simulink model "Virtual_Fuel_Air_Setpoint_Generator"  (R2016b)
settings: Solver=FixedStepDiscrete  StartTime=0.0  StopTime=inf  FixedStep=VirtFuAirSpGenr.tiSimnTiStep_C  RelTol=1e-3  EnableMultiTasking=on
settings Model: Creator=m01wolf  LastModifiedBy=bunver
settings DataIOCC: SaveFormat=StructureWithTime  SaveOutput=off  DSMLogging=off  VisualizeSimOutput=off  SaveTime=off  StateSaveName=Results  SignalLoggingName=Results
settings OptimizationCC: BlockReduction=off  ConditionallyExecuteInputs=off  LifeSpan=inf
settings DebuggingCC: AllowSymbolicDim=off  SFUnexpectedBacktrackingDiag=warning  SFNoUnconditionalDefaultTransitionDiag=warning  SFExecutionAtInitializationDiag=none
settings ModelReferenceCC: ModelReferenceNumInstancesAllowed=Single  PropagateSignalLabelsOutOfModel=off
settings GRTTargetCC: TargetLangStandard=C89/C90 (ANSI)
settings ConfigComp: CovMetricSettings=dw  CovHtmlReporting=on  CovSaveCumulativeToWorkspaceVar=on  CovSaveSingleToWorkspaceVar=on  CovExternalEMLEnable=off

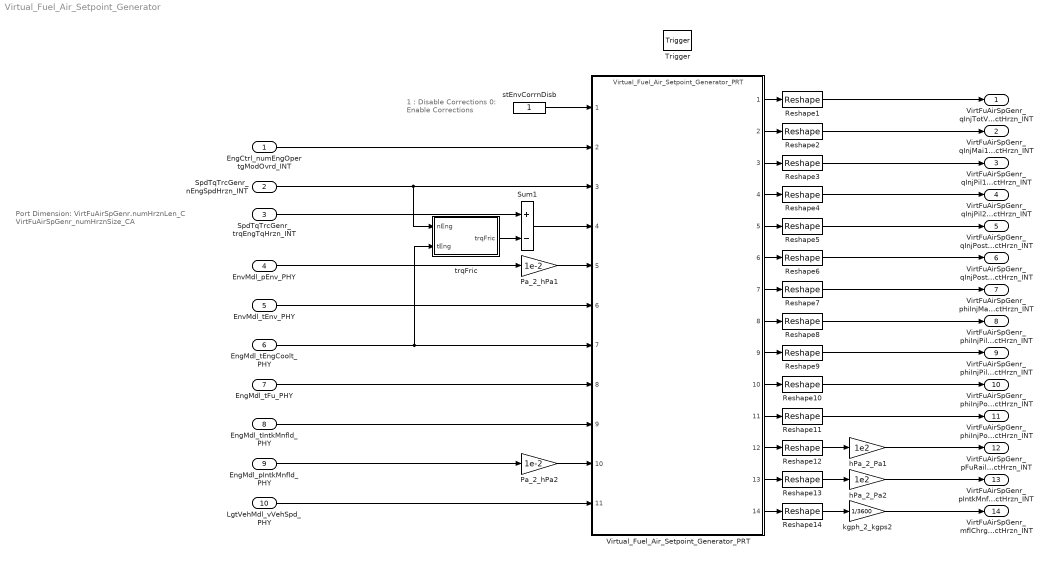
== system Virtual_Fuel_Air_Setpoint_Generator ==
  note: Port Dimension: VirtFuAirSpGenr.numHrznLen_C
      | VirtFuAirSpGenr_numHrznSize_CA
  note: 1 : Disable Corrections
      | 0: Enable Corrections
  EngCtrl_numEngOpertgModOvrd_INT : Inport
  SpdTqTrcGenr_nEngSpdHrzn_INT : Inport  Port=2  PortDimensions=VirtFuAirSpGenr_numHrznSize_CA
  SpdTqTrcGenr_trqEngTqHrzn_INT : Inport  Port=3  PortDimensions=VirtFuAirSpGenr_numHrznSize_CA
  EnvMdl_pEnv_PHY : Inport  Port=4
  EnvMdl_tEnv_PHY : Inport  Port=5
  EngMdl_tEngCoolt_PHY : Inport  Port=6
  EngMdl_tFu_PHY : Inport  Port=7
  EngMdl_tIntkMnfld_PHY : Inport  Port=8
  EngMdl_pIntkMnfld_PHY : Inport  Port=9
  LgtVehMdl_vVehSpd_PHY : Inport  Port=10
  Trigger : TriggerPort  TriggerType=function-call  VariantControl=Variant  PortDimensions=1
  Pa_2_hPa1 : Gain  Gain=1e-2
  Pa_2_hPa2 : Gain  Gain=1e-2
  Reshape{1..14} (14 alike) : Reshape
  Sum1 : Sum  Inputs=+-
      settings: AttributesFormatString=%<Name>
  Virtual_Fuel_Air_Setpoint_Generator_PRT : ModelReference  ModelNameDialog=Virtual_Fuel_Air_Setpoint_Generator_PRT.slxp  ModelReferenceVersion=1.262  CopyOfModelProtected=on
  hPa_2_Pa1 : Gain  Gain=1e2
  hPa_2_Pa2 : Gain  Gain=1e2
  kgph_2_kgps2 : Gain  Gain=1/3600
  stEnvCorrnDisb : Constant  SampleTime=-1
  trqFric : Subsystem
  VirtFuAirSpGenr_qInjTotVectHrzn_INT : Outport
  VirtFuAirSpGenr_qInjMai1VectHrzn_INT : Outport  Port=2
  VirtFuAirSpGenr_qInjPil1VectHrzn_INT : Outport  Port=3
  VirtFuAirSpGenr_qInjPil2VectHrzn_INT : Outport  Port=4
  VirtFuAirSpGenr_qInjPost1VectHrzn_INT : Outport  Port=5
  VirtFuAirSpGenr_qInjPost2VectHrzn_INT : Outport  Port=6
  VirtFuAirSpGenr_phiInjMai1VectHrzn_INT : Outport  Port=7
  VirtFuAirSpGenr_phiInjPil1VectHrzn_INT : Outport  Port=8
  VirtFuAirSpGenr_phiInjPil2VectHrzn_INT : Outport  Port=9
  VirtFuAirSpGenr_phiInjPost1VectHrzn_INT : Outport  Port=10
  VirtFuAirSpGenr_phiInjPost2VectHrzn_INT : Outport  Port=11
  VirtFuAirSpGenr_pFuRailDesVectHrzn_INT : Outport  Port=12
  VirtFuAirSpGenr_pIntkMnfldDesVectHrzn_INT : Outport  Port=13
  VirtFuAirSpGenr_mflChrgdAirDesVectHrzn_INT : Outport  Port=14
  wires:
  Virtual_Fuel_Air_Setpoint_Generator_PRT/1 -> Reshape1/1
  hPa_2_Pa1/1 -> VirtFuAirSpGenr_pFuRailDesVectHrzn_INT/1
  hPa_2_Pa2/1 -> VirtFuAirSpGenr_pIntkMnfldDesVectHrzn_INT/1
  kgph_2_kgps2/1 -> VirtFuAirSpGenr_mflChrgdAirDesVectHrzn_INT/1
  Virtual_Fuel_Air_Setpoint_Generator_PRT/2 -> Reshape2/1
  Virtual_Fuel_Air_Setpoint_Generator_PRT/3 -> Reshape3/1
  Virtual_Fuel_Air_Setpoint_Generator_PRT/4 -> Reshape4/1
  Virtual_Fuel_Air_Setpoint_Generator_PRT/5 -> Reshape5/1
  Virtual_Fuel_Air_Setpoint_Generator_PRT/6 -> Reshape6/1
  Virtual_Fuel_Air_Setpoint_Generator_PRT/7 -> Reshape7/1
  Virtual_Fuel_Air_Setpoint_Generator_PRT/8 -> Reshape8/1
  Virtual_Fuel_Air_Setpoint_Generator_PRT/9 -> Reshape9/1
  Virtual_Fuel_Air_Setpoint_Generator_PRT/10 -> Reshape10/1
  Virtual_Fuel_Air_Setpoint_Generator_PRT/11 -> Reshape11/1
  Virtual_Fuel_Air_Setpoint_Generator_PRT/12 -> Reshape12/1
  Virtual_Fuel_Air_Setpoint_Generator_PRT/13 -> Reshape13/1
  Virtual_Fuel_Air_Setpoint_Generator_PRT/14 -> Reshape14/1
  trqFric/1(trqFric) -> Sum1/2
  Reshape1/1 -> VirtFuAirSpGenr_qInjTotVectHrzn_INT/1
  Reshape2/1 -> VirtFuAirSpGenr_qInjMai1VectHrzn_INT/1
  Reshape3/1 -> VirtFuAirSpGenr_qInjPil1VectHrzn_INT/1
  Reshape4/1 -> VirtFuAirSpGenr_qInjPil2VectHrzn_INT/1
  Reshape5/1 -> VirtFuAirSpGenr_qInjPost1VectHrzn_INT/1
  Reshape6/1 -> VirtFuAirSpGenr_qInjPost2VectHrzn_INT/1
  Reshape7/1 -> VirtFuAirSpGenr_phiInjMai1VectHrzn_INT/1
  Reshape8/1 -> VirtFuAirSpGenr_phiInjPil1VectHrzn_INT/1
  Reshape9/1 -> VirtFuAirSpGenr_phiInjPil2VectHrzn_INT/1
  Reshape10/1 -> VirtFuAirSpGenr_phiInjPost1VectHrzn_INT/1
  Reshape11/1 -> VirtFuAirSpGenr_phiInjPost2VectHrzn_INT/1
  Reshape12/1 -> hPa_2_Pa1/1
  Reshape13/1 -> hPa_2_Pa2/1
  Reshape14/1 -> kgph_2_kgps2/1
  SpdTqTrcGenr_nEngSpdHrzn_INT/1 -> Virtual_Fuel_Air_Setpoint_Generator_PRT/3, trqFric/1(nEng)
  SpdTqTrcGenr_trqEngTqHrzn_INT/1 -> Sum1/1
  EnvMdl_pEnv_PHY/1 -> Pa_2_hPa1/1
  EngMdl_tEngCoolt_PHY/1 -> Virtual_Fuel_Air_Setpoint_Generator_PRT/7, trqFric/2(tEng)
  EngMdl_pIntkMnfld_PHY/1 -> Pa_2_hPa2/1
  stEnvCorrnDisb/1 -> Virtual_Fuel_Air_Setpoint_Generator_PRT/1
  EngCtrl_numEngOpertgModOvrd_INT/1 -> Virtual_Fuel_Air_Setpoint_Generator_PRT/2
  Sum1/1 -> Virtual_Fuel_Air_Setpoint_Generator_PRT/4
  Pa_2_hPa1/1 -> Virtual_Fuel_Air_Setpoint_Generator_PRT/5
  EnvMdl_tEnv_PHY/1 -> Virtual_Fuel_Air_Setpoint_Generator_PRT/6
  EngMdl_tFu_PHY/1 -> Virtual_Fuel_Air_Setpoint_Generator_PRT/8
  EngMdl_tIntkMnfld_PHY/1 -> Virtual_Fuel_Air_Setpoint_Generator_PRT/9
  Pa_2_hPa2/1 -> Virtual_Fuel_Air_Setpoint_Generator_PRT/10
  LgtVehMdl_vVehSpd_PHY/1 -> Virtual_Fuel_Air_Setpoint_Generator_PRT/11

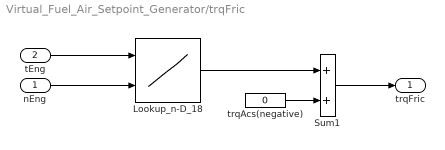
== system Virtual_Fuel_Air_Setpoint_Generator/trqFric ==
  nEng : Inport
  tEng : Inport  Port=2
  Lookup_n-D_18 : Lookup_n-D  BreakpointsForDimension1=[-30.14;-20.14;-10.14;-0.140000000000009;9.85999999999999;19.86;29.86;39.86;49.86;59.86;69.86;79.86;89.86;99.86;109.86;119.86]  BreakpointsForDimension2=[600 700 800 900 1000 1100 1200 1300 1400 1500 1600 1700 1800 1900 2000 2100]  Table=[-490 -505 -515 -520 -530 -540 -545 -550 -555 -560 -565 -570 -575 -580 -590 -600;-490 -505 -515 -520 -530 -540 -545 -550 -555 -560 -565 -570 -575 -580 -590 -600;-420 -427 -431 -433 -435 -437 -441.333343505859 -445.666656494141 -450 -455 -460 -465 -470 -500 -515 -524;-250 -277.5 -305 -309 -311 -316 -324 -335 -345 -352 -365 -379 -397 -410 -425 -450;-234 -249.25 -266.5 -271 -274 -283 -293.904754638672 -306.309509277344 -318.214294433594 -330 -342.023803710938 -355.928588867188 -370 -392.75 -415.5 -436.75;-218 -221 -228 -233 -237 -250 -263.809509277344 -277.619049072266 -291.428558349609 -304 -319.047607421875 -332.857147216797 -346.666656494141 -372.375 -393 -413.5;-199.5 -201.5 -208.5 -213 -217.5 -230 -242.904754638672 -256.809509277344 -270.714294433594 -284.619049072266 -297.523803710938 -310.928588867188 -323.333343505859 -352 -370.5 -390.25;-181 -182 -189 -193 -198 -210 -222 -236 -250 -264 -276 -289 -300 -329 -348 -367;-138 -149.199996948242 -159.399993896484 -170 -181.100006103516 -192.600006103516 -204.899993896484 -222 -236.100006103516 -246.899993896484 -263.600006103516 -277.5 -286.100006103516 -297.200012207031 -325.700012207031 -344.899993896484;-129 -138.300003051758 -147.699996948242 -157.800003051758 -168.100006103516 -179.600006103516 -191.100006103516 -207.300003051758 -223.5 -235.600006103516 -249.399993896484 -255.399993896484 -271 -284.899993896484 -310.700012207031 -321.899993896484;-117.300003051758 -128.300003051758 -138.300003051758 -148.600006103516 -159.199996948242 -164.300003051758 -179.199996948242 -196.699996948242 -216 -220.800003051758 -233.300003051758 -252 -256.799987792969 -274.5 -296.899993896484 -316.200012207031;-110.099998474121 -120.900001525879 -124.699996948242 -137.600006103516 -148.699996948242 -160 -171.699996948242 -185.800003051758 -203.100006103516 -210.899993896484 -219.800003051758 -232.899993896484 -247.699996948242 -259 -277 -295.600006103516;-108.699996948242 -114.900001525879 -122.400001525879 -130.199996948242 -135.600006103516 -150.800003051758 -162.600006103516 -177.100006103516 -193.399993896484 -202 -210.5 -223.199996948242 -235.699996948242 -249.300003051758 -268.200012207031 -286.399993896484;-104.900001525879 -109.800003051758 -115 -125.699996948242 -134.699996948242 -143.199996948242 -154.899993896484 -169.699996948242 -188.300003051758 -196.5 -205.800003051758 -218.199996948242 -230.399993896484 -244.199996948242 -263.799987792969 -282.899993896484;-101.900001525879 -102.099998474121 -112 -122 -125.5 -140.199996948242 -151.899993896484 -166.300003051758 -183.300003051758 -190.5 -200.600006103516 -213.300003051758 -221.800003051758 -238.199996948242 -257.100006103516 -275.700012207031;-96 -97 -109 -117.199996948242 -120 -131.100006103516 -140.399993896484 -156 -175 -185 -195 -207 -212 -230 -250 -268]  ExtrapMethod=Clip  UseLastTableValue=on  RndMeth=Simplest  InputSameDT=on
  Sum1 : Sum
      settings: AttributesFormatString=%<Name>
  trqAcs(negative) : Constant  Value=0  SampleTime=-1
  trqFric : Outport
  wires:
  nEng/1 -> Lookup_n-D_18/2
  tEng/1 -> Lookup_n-D_18/1
  Lookup_n-D_18/1 -> Sum1/1
  Sum1/1 -> trqFric/1
  trqAcs(negative)/1 -> Sum1/2
